simulink subsystem "PickingObj"  (R2023a)
settings: Solver=VariableStepAuto  StartTime=0.0  StopTime=10.0  RelTol=1e-3
undefined symbols (not defined in the file): Environment
libraries: nesl_utility x2, sm_lib x1
settings Model: Creator=Dell  LastModifiedBy=danie

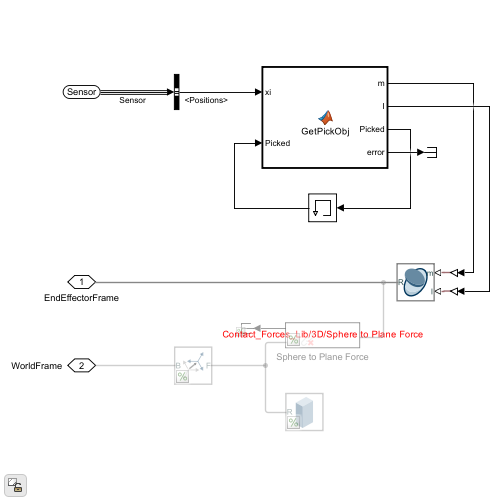
[thumbnail: Simulink's stored preview of the top-level diagram]
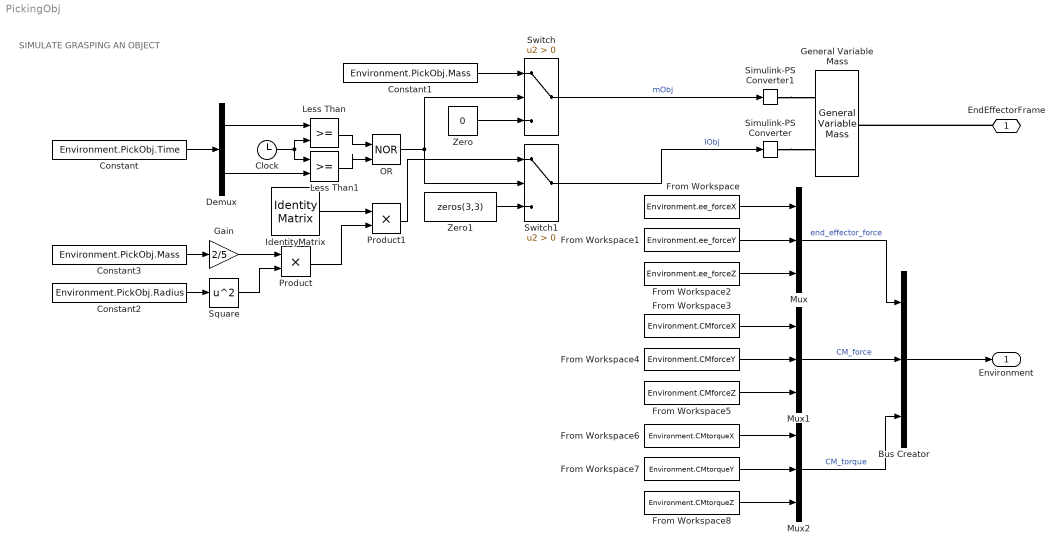
== system PickingObj ==
  note: SIMULATE GRASPING AN OBJECT
  Bus Creator : BusCreator  Inputs=3
  Clock : Clock
  Constant : Constant  Value=Environment.PickObj.Time
  Constant1 : Constant  Value=Environment.PickObj.Mass
  Constant2 : Constant  Value=Environment.PickObj.Radius
  Constant3 : Constant  Value=Environment.PickObj.Mass
  Demux : Demux  Outputs=2
  From Workspace : FromWorkspace  VariableName=Environment.ee_forceX  SampleTime=0.01
  From Workspace1 : FromWorkspace  VariableName=Environment.ee_forceY  SampleTime=0.01
  From Workspace2 : FromWorkspace  VariableName=Environment.ee_forceZ  SampleTime=0.01
  From Workspace3 : FromWorkspace  VariableName=Environment.CMforceX  SampleTime=0.01
  From Workspace4 : FromWorkspace  VariableName=Environment.CMforceY  SampleTime=0.01
  From Workspace5 : FromWorkspace  VariableName=Environment.CMforceZ  SampleTime=0.01
  From Workspace6 : FromWorkspace  VariableName=Environment.CMtorqueX  SampleTime=0.01
  From Workspace7 : FromWorkspace  VariableName=Environment.CMtorqueY  SampleTime=0.01
  From Workspace8 : FromWorkspace  VariableName=Environment.CMtorqueZ  SampleTime=0.01
  Gain : Gain  Gain=2/5
  General Variable Mass : sm_lib/Body Elements/Variable Mass/General Variable Mass  VariableInertiaType=Custom  MassType=TimeVarying  Mass=1  MassUnits=kg  CenterOfMassType=Constant  CenterOfMass=[0 0 0]  CenterOfMassUnits=m  InertiaMatrixType=TimeVarying  MomentsOfInertia=[1 1 1]  MomentsOfInertiaUnits=kg*m^2  ProductsOfInertia=[0 0 0]  ProductsOfInertiaUnits=kg*m^2  GraphicType=InertiaEllipsoid  MarkerShape=Sphere  MarkerSize=10  GraphicVisPropType=SimpleVisualProperties  GraphicDiffuseColor=[1 0 0]  GraphicSpecularColor=[0.5 0.5 0.5 1.0]  GraphicAmbientColor=[0.15 0.15 0.15 1.0]  GraphicEmissiveColor=[0.0 0.0 0.0 1.0]  GraphicShininess=75  GraphicOpacity=1.0
  IdentityMatrix : IdentityMatrix  OutputDimensions=3
  Less Than : RelationalOperator  OutDataTypeStr=boolean  RndMeth=Simplest  InputSameDT=off
  Less Than1 : RelationalOperator  OutDataTypeStr=boolean  RndMeth=Simplest  InputSameDT=off
  Mux : Mux  Inputs=3
  Mux1 : Mux  Inputs=3
  Mux2 : Mux  Inputs=3
  OR : Logic  Operator=NOR  IconShape=distinctive  AllPortsSameDT=off  OutDataTypeStr=boolean
  Product : Product
  Product1 : Product
  Simulink-PS Converter : nesl_utility/Simulink-PS Converter  PhysicalDomain=network_engine_domain  SubClassName=ps_input  LeftPortType=input  RightPortType=output  PseudoPeriodic=off  Frequencies=[]  NoiseDistribution=none  NoiseParameters=[]  Unit=1  AffineConversion=off  FilteringAndDerivatives=provide  SimscapeFilterOrder=1  InputFilterTimeConstant=0.001  UdotUserProvided=0
  Simulink-PS Converter1 : nesl_utility/Simulink-PS Converter  PhysicalDomain=network_engine_domain  SubClassName=ps_input  LeftPortType=input  RightPortType=output  PseudoPeriodic=off  Frequencies=[]  NoiseDistribution=none  NoiseParameters=[]  Unit=1  AffineConversion=off  FilteringAndDerivatives=provide  SimscapeFilterOrder=1  InputFilterTimeConstant=0.001  UdotUserProvided=0
  Square : Math  Operator=square
  Switch : Switch  Criteria=u2 > Threshold  SaturateOnIntegerOverflow=off  InputSameDT=off
  Switch1 : Switch  Criteria=u2 > Threshold  SaturateOnIntegerOverflow=off  InputSameDT=off
  Zero : Constant  Value=0  OutDataTypeStr=Inherit: Inherit via back propagation
  Zero1 : Constant  Value=zeros(3,3)  OutDataTypeStr=Inherit: Inherit via back propagation
  EndEffectorFrame : PMIOPort  Side=Left
  Environment : Outport
  wires:
  Switch1/1 -> Simulink-PS Converter/1  "IObj"
  Switch/1 -> Simulink-PS Converter1/1  "mObj"
  From Workspace/1 -> Mux/1
  From Workspace1/1 -> Mux/2
  From Workspace2/1 -> Mux/3
  Bus Creator/1 -> Environment/1
  Mux/1 -> Bus Creator/1  "end_effector_force"
  From Workspace3/1 -> Mux1/1
  From Workspace4/1 -> Mux1/2
  From Workspace5/1 -> Mux1/3
  Mux1/1 -> Bus Creator/2  "CM_force"
  From Workspace6/1 -> Mux2/1
  From Workspace7/1 -> Mux2/2
  From Workspace8/1 -> Mux2/3
  Mux2/1 -> Bus Creator/3  "CM_torque"
  Constant1/1 -> Switch/1
  Constant2/1 -> Square/1
  Constant/1 -> Demux/1
  Demux/1 -> Less Than/1
  Clock/1 -> Less Than1/1, Less Than/2
  Demux/2 -> Less Than1/2
  Less Than/1 -> OR/1
  Less Than1/1 -> OR/2
  OR/1 -> Switch/2, Switch1/2
  Zero/1 -> Switch/3
  Constant3/1 -> Gain/1
  Gain/1 -> Product/1
  Square/1 -> Product/2
  IdentityMatrix/1 -> Product1/1
  Product/1 -> Product1/2
  Product1/1 -> Switch1/1
  Zero1/1 -> Switch1/3
  connections:
  EndEffectorFrame/RConn1 -- General Variable Mass/RConn1
  Simulink-PS Converter/RConn1 -- General Variable Mass/LConn2
  Simulink-PS Converter1/RConn1 -- General Variable Mass/LConn1
